simulink model "machine3_step_comp"  (R2023a)
settings: Solver=FixedStepAuto  StartTime=0.0  StopTime=10.0  RelTol=1e-3
settings Model: Creator=andre  LastModifiedBy=andre

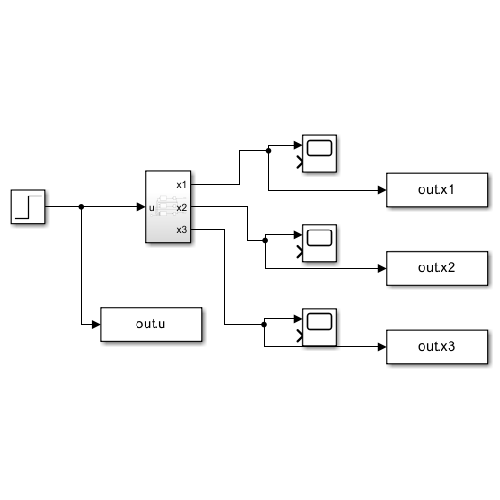
[thumbnail: Simulink's stored preview of the top-level diagram]
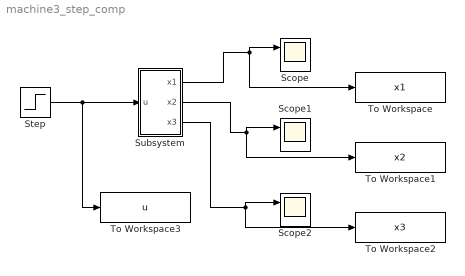
== system machine3_step_comp ==
  Scope : Scope  NumInputPorts=2
  Scope1 : Scope  NumInputPorts=2
  Scope2 : Scope  NumInputPorts=2
  Step : Step  SampleTime=0
  Subsystem : Subsystem
  To Workspace : ToWorkspace  VariableName=x1  SaveFormat=Structure With Time  SampleTime=-1
  To Workspace1 : ToWorkspace  VariableName=x2  SaveFormat=Structure With Time  SampleTime=-1
  To Workspace2 : ToWorkspace  VariableName=x3  SaveFormat=Structure With Time  SampleTime=-1
  To Workspace3 : ToWorkspace  VariableName=u  SaveFormat=Structure With Time  SampleTime=-1
  wires:
  Step/1 -> To Workspace3/1, Subsystem/1(u)
  Subsystem/1(x1) -> To Workspace/1, Scope/1
  Subsystem/2(x2) -> To Workspace1/1, Scope1/1
  Subsystem/3(x3) -> To Workspace2/1, Scope2/1

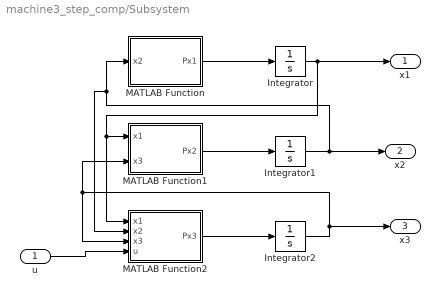
== system machine3_step_comp/Subsystem ==
  u : Inport
  Integrator : Integrator  InitialCondition=1
  Integrator1 : Integrator  InitialCondition=1
  Integrator2 : Integrator  InitialCondition=1
  MATLAB Function : MATLAB Function  TreatAsAtomicUnit=on
  MATLAB Function1 : MATLAB Function  TreatAsAtomicUnit=on
  MATLAB Function2 : MATLAB Function  TreatAsAtomicUnit=on
  x1 : Outport
  x2 : Outport  Port=2
  x3 : Outport  Port=3
  wires:
  MATLAB Function/1(Px1) -> Integrator/1
  Integrator2/1 -> x3/1, MATLAB Function2/3(x3), MATLAB Function1/2(x3)
  Integrator1/1 -> x2/1, MATLAB Function/1(x2), MATLAB Function2/2(x2)
  u/1 -> MATLAB Function2/4(u)
  MATLAB Function2/1(Px3) -> Integrator2/1
  Integrator/1 -> x1/1, MATLAB Function2/1(x1), MATLAB Function1/1(x1)
  MATLAB Function1/1(Px2) -> Integrator1/1

== matlab function machine3_step_comp/Subsystem/MATLAB Function1 ==
  data: x1 input; Px2 output; x3 input
function Px2 = fcn(x1,x3)

gc = 9.81^(-2);
c = 1.24*10^(-2);
m = 11.87;

Px2 = gc-(c/m)*(x3/x1)^2;

== matlab function machine3_step_comp/Subsystem/MATLAB Function ==
  data: x2 input; Px1 output
function Px1 = fcn(x2)

Px1 = x2;

== matlab function machine3_step_comp/Subsystem/MATLAB Function2 ==
  data: x1 input; Px3 output; x2 input; x3 input; u input
function Px3 = fcn(x1,x2,x3,u)

R = 28.7;
L = 0.65;
C = 1.24*10^(-2);

Px3 = (-R/L)*x3 + ((2*C)/L)*((x2*x3)/(x1*2)) + (u/L);
